simulink model "Comparison"  (R2020a)
settings: Solver=VariableStepAuto  StartTime=0.0  StopTime=10.0  RelTol=1e-3
undefined symbols (not defined in the file or in its folder): deg, InitialCondition, rad, s
libraries: aerolibconvert2 x9
settings Model: Creator=DELL  LastModifiedBy=DELL

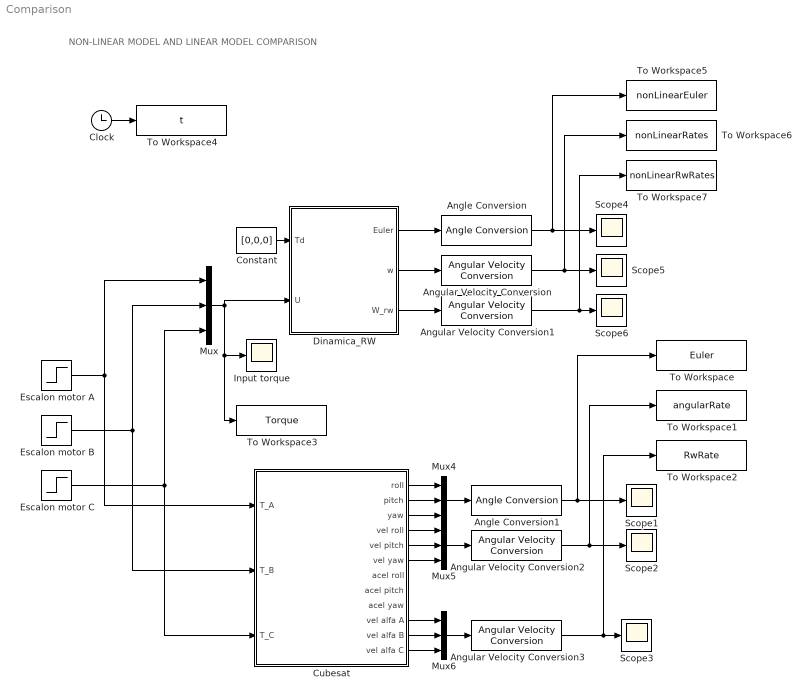
== system Comparison ==
  note: NON-LINEAR MODEL AND LINEAR MODEL COMPARISON
  Angle Conversion : aerolibconvert2/Angle Conversion  IU=rad  OU=deg
  Angle Conversion1 : aerolibconvert2/Angle Conversion  IU=deg  OU=rad
  Angular Velocity Conversion{,1..3} (4 alike) : aerolibconvert2/Angular Velocity Conversion  IU=rad/s  OU=rpm
  Clock : Clock
  Constant : Constant  Value=[0,0,0]
  Cubesat : Subsystem  mask{Iw=1.604*10^-5, Ib=4.26*10^-3, mw=0.02, lw=0.092, Bw=0.0035*10^-3}
      mask prompts: Iw "Momento de inercia de rueda de reacción"; Ib "Momento de inercia de CubeSat"; mw "Masa de Rueda de reacción"; lw "Longitud de CM de CubeSat a eje de rueda"; Bw "Coeficiente de friccion"
  Dinamica_RW : Subsystem  mask{I=[8.46,8.46,8.46,1.1,1.5,1.6]*10^(-3), Ang=[0,0,0], W=[0,0,0], Wrw=[0,0,0], dimensiones=[0.015,0.025,0.043]}
      mask prompts: I "[Ix,Iy,Iz,Ixy,Ixz,Iyz] :"; Ang "[roll,pitch,yaw]:"; W "[Wx,Wy,Wz]"; Wrw "[Wrwx,Wrwy,Wrwz]"; dimensiones "[Ancho,Masa,Radio]:"
      mask TypeOptions I: I/Value
      mask TypeOptions Ang: Ang/Value
      mask TypeOptions W: W/Value
      mask TypeOptions Wrw: Wrw/Value
      mask TypeOptions dimensiones: dimentions/Value
      mask DialogControl Container3 Prompt: Tensor de Inercia
      mask DialogControl Container2 Prompt: Condiciones iniciales
      mask DialogControl Container4 Prompt: Ruedas de Reacción:
      mask DialogControl Control1 Prompt: Dimensiones:
  Escalon motor A : Step  Before=0.007  After=0  SampleTime=0.01
  Escalon motor B : Step  After=0  SampleTime=0.01
  Escalon motor C : Step  After=0  SampleTime=0.01
  Input torque : Scope
  Mux{,4..6} (4 alike) : Mux  Inputs=3
  Scope{1..6} (6 alike) : Scope
  To Workspace : ToWorkspace  VariableName=Euler  SampleTime=-1
  To Workspace1 : ToWorkspace  VariableName=angularRate  SampleTime=-1
  To Workspace2 : ToWorkspace  VariableName=RwRate  SampleTime=-1
  To Workspace3 : ToWorkspace  VariableName=Torque  SampleTime=-1
  To Workspace4 : ToWorkspace  VariableName=t  SampleTime=-1
  To Workspace5 : ToWorkspace  VariableName=nonLinearEuler  SampleTime=-1
  To Workspace6 : ToWorkspace  VariableName=nonLinearRates  SampleTime=-1
  To Workspace7 : ToWorkspace  VariableName=nonLinearRwRates  SampleTime=-1
  wires:
  Clock/1 -> To Workspace4/1
  Angular Velocity Conversion2/1 -> Scope2/1, To Workspace1/1
  Mux/1 -> To Workspace3/1, Input torque/1, Dinamica_RW/2(U)
  Escalon motor C/1 -> Cubesat/3(T_C), Mux/3
  Escalon motor A/1 -> Cubesat/1(T_A), Mux/1
  Angular Velocity Conversion3/1 -> Scope3/1, To Workspace2/1
  Angle Conversion1/1 -> Scope1/1, To Workspace/1
  Escalon motor B/1 -> Cubesat/2(T_B), Mux/2
  Constant/1 -> Dinamica_RW/1(Td)
  Dinamica_RW/1(Euler) -> Angle Conversion/1
  Dinamica_RW/2("w ") -> Angular Velocity Conversion/1
  Dinamica_RW/3(W_rw) -> Angular Velocity Conversion1/1
  Angle Conversion/1 -> To Workspace5/1, Scope4/1
  Angular Velocity Conversion/1 -> Scope5/1, To Workspace6/1
  Angular Velocity Conversion1/1 -> To Workspace7/1, Scope6/1
  Cubesat/2(pitch) -> Mux4/2
  Cubesat/1(roll) -> Mux4/1
  Cubesat/3(yaw) -> Mux4/3
  Cubesat/4(vel roll) -> Mux5/1
  Cubesat/5(vel pitch) -> Mux5/2
  Cubesat/6(vel yaw) -> Mux5/3
  Cubesat/10(vel alfa A) -> Mux6/1
  Cubesat/11(vel alfa B) -> Mux6/2
  Cubesat/12(vel alfa C) -> Mux6/3
  Mux4/1 -> Angle Conversion1/1
  Mux5/1 -> Angular Velocity Conversion2/1
  Mux6/1 -> Angular Velocity Conversion3/1

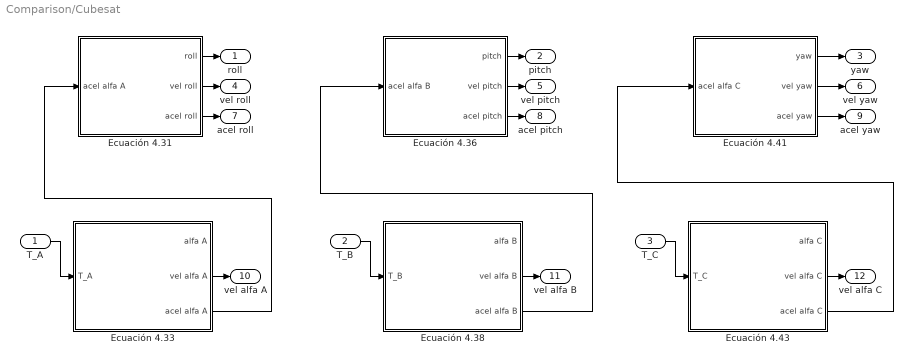
== system Comparison/Cubesat ==
  T_A : Inport
  T_B : Inport  Port=2
  T_C : Inport  Port=3
  Ecuación 4.31 : Subsystem
  Ecuación 4.33 : Subsystem
  Ecuación 4.36 : Subsystem
  Ecuación 4.38 : Subsystem
  Ecuación 4.41 : Subsystem
  Ecuación 4.43 : Subsystem
  roll : Outport
  pitch : Outport  Port=2
  yaw : Outport  Port=3
  vel roll : Outport  Port=4
  vel pitch : Outport  Port=5
  vel yaw : Outport  Port=6
  acel roll : Outport  Port=7
  acel pitch : Outport  Port=8
  acel yaw : Outport  Port=9
  vel alfa A : Outport  Port=10
  vel alfa B : Outport  Port=11
  vel alfa C : Outport  Port=12
  wires:
  Ecuación 4.41/2(vel yaw) -> vel yaw/1
  Ecuación 4.41/3(acel yaw) -> acel yaw/1
  Ecuación 4.41/1(yaw) -> yaw/1
  Ecuación 4.33/3(acel alfa A) -> Ecuación 4.31/1(acel alfa A)
  Ecuación 4.43/3(acel alfa C) -> Ecuación 4.41/1(acel alfa C)
  Ecuación 4.33/2(vel alfa A) -> vel alfa A/1
  Ecuación 4.36/2(vel pitch) -> vel pitch/1
  T_B/1 -> Ecuación 4.38/1(T_B)
  T_A/1 -> Ecuación 4.33/1(T_A)
  Ecuación 4.43/2(vel alfa C) -> vel alfa C/1
  Ecuación 4.31/1(roll) -> roll/1
  Ecuación 4.36/1(pitch) -> pitch/1
  Ecuación 4.31/2(vel roll) -> vel roll/1
  Ecuación 4.31/3(acel roll) -> acel roll/1
  Ecuación 4.38/2(vel alfa B) -> vel alfa B/1
  Ecuación 4.36/3(acel pitch) -> acel pitch/1
  T_C/1 -> Ecuación 4.43/1(T_C)
  Ecuación 4.38/3(acel alfa B) -> Ecuación 4.36/1(acel alfa B)

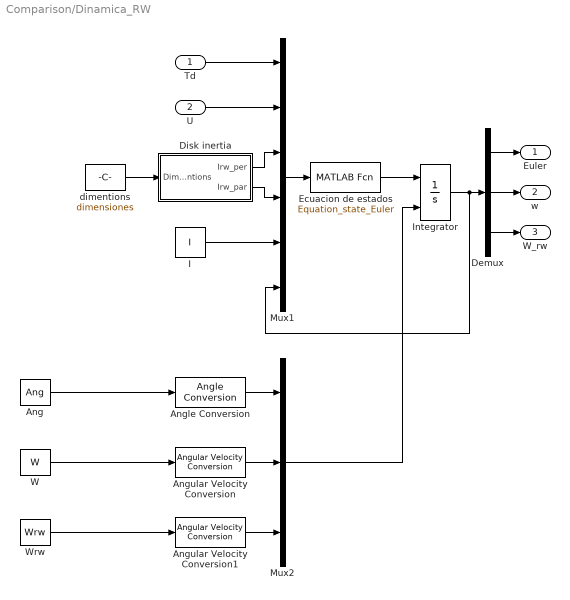
== system Comparison/Dinamica_RW ==
  Td : Inport
  U : Inport  Port=2
  Ang : Constant  Value=Ang
  Angle Conversion : aerolibconvert2/Angle Conversion  IU=deg  OU=rad
  Angular Velocity Conversion : aerolibconvert2/Angular Velocity Conversion  IU=deg/s  OU=rad/s
  Angular Velocity Conversion1 : aerolibconvert2/Angular Velocity Conversion  IU=deg/s  OU=rad/s
  Demux : Demux  Outputs=3
  Disk inertia : Subsystem
  Ecuacion de estados : MATLABFcn  MATLABFcn=Equation_state_Euler
  I : Constant  Value=I
  Integrator : Integrator  InitialConditionSource=external  InitialCondition=InitialCondition
  Mux1 : Mux  Inputs=6
  Mux2 : Mux  Inputs=3
  W : Constant  Value=W
  Wrw : Constant  Value=Wrw
  dimentions : Constant  Value=dimensiones
  Euler : Outport
  "w " : Outport  Port=2
  W_rw : Outport  Port=3
  wires:
  Disk inertia/2(Irw_par) -> Mux1/4
  Disk inertia/1(Irw_per) -> Mux1/3
  dimentions/1 -> Disk inertia/1(Dimentions)
  W/1 -> Angular Velocity Conversion/1
  Integrator/1 -> Demux/1, Mux1/6
  Angle Conversion/1 -> Mux2/1
  Wrw/1 -> Angular Velocity Conversion1/1
  Ang/1 -> Angle Conversion/1
  Angular Velocity Conversion/1 -> Mux2/2
  Angular Velocity Conversion1/1 -> Mux2/3
  Mux2/1 -> Integrator/2
  I/1 -> Mux1/5
  U/1 -> Mux1/2
  Mux1/1 -> Ecuacion de estados/1
  Ecuacion de estados/1 -> Integrator/1
  Td/1 -> Mux1/1
  Demux/2 -> "w "/1
  Demux/3 -> W_rw/1
  Demux/1 -> Euler/1

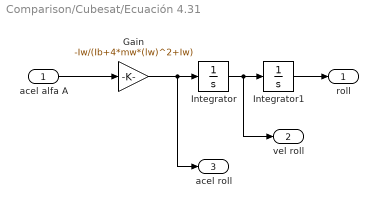
== system Comparison/Cubesat/Ecuación 4.31 ==
  acel alfa A : Inport
  Gain : Gain  Gain=-Iw/(Ib+4*mw*(lw)^2+Iw)
  Integrator : Integrator
  Integrator1 : Integrator
  roll : Outport
  vel roll : Outport  Port=2
  acel roll : Outport  Port=3
  wires:
  acel alfa A/1 -> Gain/1
  Gain/1 -> acel roll/1, Integrator/1
  Integrator/1 -> vel roll/1, Integrator1/1
  Integrator1/1 -> roll/1

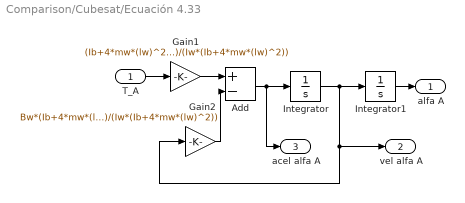
== system Comparison/Cubesat/Ecuación 4.33 ==
  T_A : Inport
  Add : Sum  Inputs=+-
  Gain1 : Gain  Gain=(Ib+4*mw*(lw)^2+Iw)/(Iw*(Ib+4*mw*(lw)^2))
  Gain2 : Gain  Gain=Bw*(Ib+4*mw*(lw)^2+Iw)/(Iw*(Ib+4*mw*(lw)^2))
  Integrator : Integrator
  Integrator1 : Integrator
  alfa A : Outport
  vel alfa A : Outport  Port=2
  acel alfa A : Outport  Port=3
  wires:
  Integrator/1 -> Integrator1/1, vel alfa A/1, Gain2/1
  T_A/1 -> Gain1/1
  Gain2/1 -> Add/2
  Add/1 -> Integrator/1, acel alfa A/1
  Gain1/1 -> Add/1
  Integrator1/1 -> alfa A/1

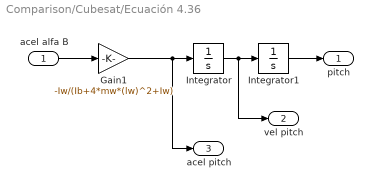
== system Comparison/Cubesat/Ecuación 4.36 ==
  acel alfa B : Inport
  Gain1 : Gain  Gain=-Iw/(Ib+4*mw*(lw)^2+Iw)
  Integrator : Integrator
  Integrator1 : Integrator
  pitch : Outport
  vel pitch : Outport  Port=2
  acel pitch : Outport  Port=3
  wires:
  Gain1/1 -> acel pitch/1, Integrator/1
  Integrator/1 -> vel pitch/1, Integrator1/1
  acel alfa B/1 -> Gain1/1
  Integrator1/1 -> pitch/1

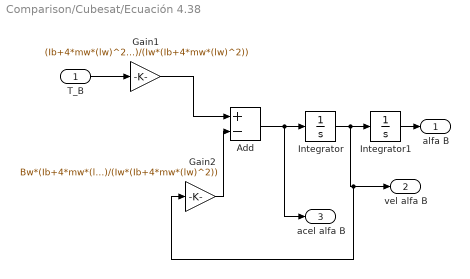
== system Comparison/Cubesat/Ecuación 4.38 ==
  T_B : Inport
  Add : Sum  Inputs=+-
  Gain1 : Gain  Gain=(Ib+4*mw*(lw)^2+Iw)/(Iw*(Ib+4*mw*(lw)^2))
  Gain2 : Gain  Gain=Bw*(Ib+4*mw*(lw)^2+Iw)/(Iw*(Ib+4*mw*(lw)^2))
  Integrator : Integrator
  Integrator1 : Integrator
  alfa B : Outport
  vel alfa B : Outport  Port=2
  acel alfa B : Outport  Port=3
  wires:
  Integrator/1 -> Gain2/1, vel alfa B/1, Integrator1/1
  T_B/1 -> Gain1/1
  Gain2/1 -> Add/2
  Add/1 -> acel alfa B/1, Integrator/1
  Gain1/1 -> Add/1
  Integrator1/1 -> alfa B/1

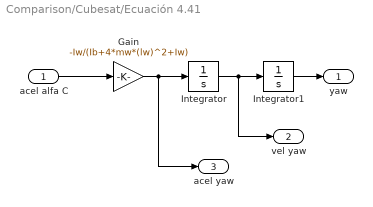
== system Comparison/Cubesat/Ecuación 4.41 ==
  acel alfa C : Inport
  Gain : Gain  Gain=-Iw/(Ib+4*mw*(lw)^2+Iw)
  Integrator : Integrator
  Integrator1 : Integrator
  yaw : Outport
  vel yaw : Outport  Port=2
  acel yaw : Outport  Port=3
  wires:
  Gain/1 -> Integrator/1, acel yaw/1
  Integrator/1 -> Integrator1/1, vel yaw/1
  acel alfa C/1 -> Gain/1
  Integrator1/1 -> yaw/1

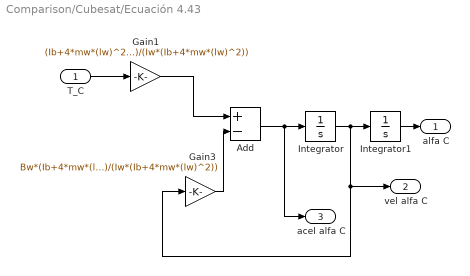
== system Comparison/Cubesat/Ecuación 4.43 ==
  T_C : Inport
  Add : Sum  Inputs=+-
  Gain1 : Gain  Gain=(Ib+4*mw*(lw)^2+Iw)/(Iw*(Ib+4*mw*(lw)^2))
  Gain3 : Gain  Gain=Bw*(Ib+4*mw*(lw)^2+Iw)/(Iw*(Ib+4*mw*(lw)^2))
  Integrator : Integrator
  Integrator1 : Integrator
  alfa C : Outport
  vel alfa C : Outport  Port=2
  acel alfa C : Outport  Port=3
  wires:
  T_C/1 -> Gain1/1
  Gain3/1 -> Add/2
  Add/1 -> acel alfa C/1, Integrator/1
  Gain1/1 -> Add/1
  Integrator1/1 -> alfa C/1
  Integrator/1 -> Gain3/1, vel alfa C/1, Integrator1/1

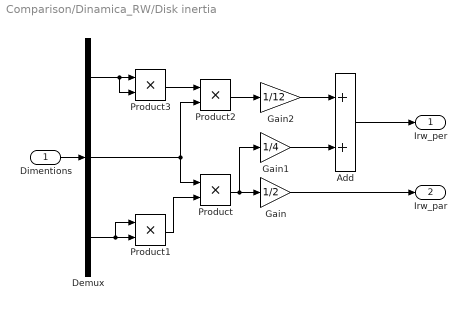
== system Comparison/Dinamica_RW/Disk inertia ==
  Dimentions : Inport
  Add : Sum
  Demux : Demux  Outputs=3
  Gain : Gain  Gain=1/2
  Gain1 : Gain  Gain=1/4
  Gain2 : Gain  Gain=1/12
  Product{,1..3} (4 alike) : Product
  Irw_per : Outport
  Irw_par : Outport  Port=2
  wires:
  Demux/3 -> Product1/2, Product1/1
  Dimentions/1 -> Demux/1
  Demux/2 -> Product2/2, Product/1
  Product2/1 -> Gain2/1
  Demux/1 -> Product3/1, Product3/2
  Gain/1 -> Irw_par/1
  Product1/1 -> Product/2
  Gain1/1 -> Add/2
  Add/1 -> Irw_per/1
  Product/1 -> Gain/1, Gain1/1
  Gain2/1 -> Add/1
  Product3/1 -> Product2/1
